simulink model "BFE_TestHarness"  (Simulink 8.6)
settings: Solver=FixedStepDiscrete  StartTime=0.0  StopTime=3  FixedStep=Ts  RelTol=1e-3
PreLoadFcn:
  | addpath('MBD_Tests')
  | 
  | load('Workspace\EnvVar.mat')
  | run('MBD_Tests\MBD_tests_init.m')
  | if exist('tl_preloadfcn','file'), tl_preloadfcn(gcs,402); end
PostLoadFcn:
  | if exist('tl_postloadfcn','file'), tl_postloadfcn(gcs,402); end
InitFcn:
  | if exist('tlds_init','file'), tlds_init(gcs); end
StartFcn:
  | if exist('tlds_start','file'), tlds_start(gcs); end
StopFcn:
  | if exist('tlds_stop','file'), tlds_stop(gcs); end
undefined symbols (not defined in the file): ddv, Ts, u2, u3, u4
libraries: tllib x11, simulink x8, LIB_TF_G_111 x2, LIB_TF_G_12_StepControl x2, LIB_TF_G_112 x1, LIB_TF_G_113 x1
(part 4 of 17)

== system BFE_TestHarness/BFE_AC_BeltFunctionExecution/Subsystem/BFE_AC_BeltFunctionExecution/BFE_AC_BeltFunctionExecution/BFE_runExecuteEmergencyBrakingSequence/Idle State ==
  s16MotorPowerOrder : Inport
  Action Port : ActionPort  ActionType=else
  BFE_MIL_MBD : Constant  RequirementInfo={} %GIDa_d04f2b34_a89a_4659_8327_de322dda7124  Value=ddv('BFE/BFE_MIL_MBD')  mask(TL_Constant){data={'output',{'variable','BFE/BFE_MIL_MBD'},'date',735951.66860642366}}
      settings: CopyFcn=if exist('tl_reset_reviewflag','file')==2,tl_reset_reviewflag(gcbh);end  DeleteFcn=if exist('delete_tlblock','file')==2,delete_tlblock(gcbh);end  NameChangeFcn=if exist('rename_tlblock','file')==2,rename_tlblock(gcbh);end  OpenFcn=if exist('tl_open_blockdlg','file')==2,tl_open_blockdlg(gcbh);else,open_system(gcbh,'parameter');end
      mask Help: eval(['if exist(''tl_online_help'',''file'') == 2, tl_online_help(''Topic'',''TL_Constant''),else, web([''jar:file:///'',matlabroot,''/help/toolbox/simulink/help.jar!/slref/' lower(get_param(gcbh,'Blocktype')) '.html''], ''-helpbrowser''),end'])
      mask Display: plot([-0.05, 1.05, NaN, -0.05, 1.05],[.01, .01, NaN, .99, .99])
  BusCreator : BusCreator  Inputs=2
  Constant : Constant  Value=256  OutDataTypeStr=int16  mask(TL_Constant){data={'date',735951.66860605322}}
      settings: CopyFcn=if exist('tl_reset_reviewflag','file')==2,tl_reset_reviewflag(gcbh);end  DeleteFcn=if exist('delete_tlblock','file')==2,delete_tlblock(gcbh);end  NameChangeFcn=if exist('rename_tlblock','file')==2,rename_tlblock(gcbh);end  OpenFcn=if exist('tl_open_blockdlg','file')==2,tl_open_blockdlg(gcbh);else,open_system(gcbh,'parameter');end
      mask Help: eval(['if exist(''tl_online_help'',''file'') == 2, tl_online_help(''Topic'',''TL_Constant''),else, web([''jar:file:///'',matlabroot,''/help/toolbox/simulink/help.jar!/slref/' lower(get_param(gcbh,'Blocktype')) '.html''], ''-helpbrowser''),end'])
      mask Display: plot([-0.05, 1.05, NaN, -0.05, 1.05],[.01, .01, NaN, .99, .99])
  Data Type Conversion : DataTypeConversion
  If Action Subsystem : Subsystem  RequirementInfo={} %GIDa_d4ad1bcd_a704_4ece_a76e_501b1194cc02  TreatAsAtomicUnit=on
  KUC_ZERO1 : Constant  RequirementInfo={} %GIDa_d1c1a169_18d8_4d2e_970c_33d0bcd7c074  Value=ddv('Common/KU16_ZERO')  mask(TL_Constant){data={'output',{'variable','Common/KU16_ZERO'},'date',735951.66860510421}}
      settings: CopyFcn=if exist('tl_reset_reviewflag','file')==2,tl_reset_reviewflag(gcbh);end  DeleteFcn=if exist('delete_tlblock','file')==2,delete_tlblock(gcbh);end  NameChangeFcn=if exist('rename_tlblock','file')==2,rename_tlblock(gcbh);end  OpenFcn=if exist('tl_open_blockdlg','file')==2,tl_open_blockdlg(gcbh);else,open_system(gcbh,'parameter');end
      mask Help: eval(['if exist(''tl_online_help'',''file'') == 2, tl_online_help(''Topic'',''TL_Constant''),else, web([''jar:file:///'',matlabroot,''/help/toolbox/simulink/help.jar!/slref/' lower(get_param(gcbh,'Blocktype')) '.html''], ''-helpbrowser''),end'])
      mask Display: plot([-0.05, 1.05, NaN, -0.05, 1.05],[.01, .01, NaN, .99, .99])
  Preprocessor IF : If  RequirementInfo={} %GIDa_7af2dae5_defd_43bb_b43b_d22b8c3639ae  IfExpression=u1  ShowElse=off  mask(TL_PreProcessorIf){data={'mode',2,'date',735951.6686047801}}
      settings: DeleteFcn=if exist('delete_tlblock','file')==2,delete_tlblock(gcbh);end  NameChangeFcn=if exist('rename_tlblock','file')==2,rename_tlblock(gcbh);end  OpenFcn=if exist('tl_open_blockdlg','file')==2,tl_open_blockdlg(gcbh);else,open_system(gcbh,'parameter');end
      mask Help: eval(['if exist(''tl_online_help'',''file'') == 2, tl_online_help(''Topic'',''TL_PreProcessorIf''),else, web([''jar:file:///'',matlabroot,''/help/toolbox/simulink/help.jar!/slref/' lower(get_param(gcbh,'Blocktype')) '.html''], ''-helpbrowser''),end'])
      mask Display:
      | plot([-0.05, 1.05, NaN, -0.05, 1.05],[.01, .01, NaN, .99, .99])
      | 
      | port_label('input', 1, 'u1')
      | port_label('output',1,'#ifdef u1');
  Saturation : Saturate  UpperLimit=ddv('Common/KS16_ZERO')  LowerLimit=ddv('BFE/KS16_PWM_MIN_BTN')  mask(TL_Saturate){data={'output',{'name','s16SaturatedPowerOrder'},'lowerlimit',{'variable','BFE/KS16_PWM_MIN_BTN'},'upperlimit',{'variable','Common/KS16_ZERO'},'date',735951.66860453703}}
      settings: CopyFcn=if exist('tl_reset_reviewflag','file')==2,tl_reset_reviewflag(gcbh);end  DeleteFcn=if exist('delete_tlblock','file')==2,delete_tlblock(gcbh);end  NameChangeFcn=if exist('rename_tlblock','file')==2,rename_tlblock(gcbh);end  OpenFcn=if exist('tl_open_blockdlg','file')==2,tl_open_blockdlg(gcbh);else,open_system(gcbh,'parameter');end
      mask Help: eval(['if exist(''tl_online_help'',''file'') == 2, tl_online_help(''Topic'',''TL_Saturate''),else, web([''jar:file:///'',matlabroot,''/help/toolbox/simulink/help.jar!/slref/' lower(get_param(gcbh,'Blocktype')) '.html''], ''-helpbrowser''),end'])
      mask Display: plot([-0.05, 1.05, NaN, -0.05, 1.05],[.01, .01, NaN, .99, .99])
  Src : Subsystem
  Sum : Sum  mask(TL_Sum){data={'output',{'name','s16UnstaturatedPowerOrder'},'date',735951.66860350699}}
      settings: CopyFcn=if exist('tl_reset_reviewflag','file')==2,tl_reset_reviewflag(gcbh);end  DeleteFcn=if exist('delete_tlblock','file')==2,delete_tlblock(gcbh);end  NameChangeFcn=if exist('rename_tlblock','file')==2,rename_tlblock(gcbh);end  OpenFcn=if exist('tl_open_blockdlg','file')==2,tl_open_blockdlg(gcbh);else,open_system(gcbh,'parameter');end
      mask Help: eval(['if exist(''tl_online_help'',''file'') == 2, tl_online_help(''Topic'',''TL_Sum''),else, web([''jar:file:///'',matlabroot,''/help/toolbox/simulink/help.jar!/slref/' lower(get_param(gcbh,'Blocktype')) '.html''], ''-helpbrowser''),end'])
      mask Display: plot([-0.05, 1.05, NaN, -0.05, 1.05],[.01, .01, NaN, .99, .99])
  SSCP_pclMotorPowerOrder_SetPowerOrder : Outport  mask(TL_BusOutport){data={'#autoscaling',2,'#message',2,'#output',2,'#logdata',2,'signals',{{'',{'s16MotorPowerOrder';'u16BoostDutyCycle'}}},'autosar',{'useautosarcommunication',1,'kind',4,'clientserverport','pclMotor_P','operation','SetPowerOrder'},'date',736301.71276452544}}
      settings: CopyFcn=if exist('tl_reset_reviewflag','file')==2,tl_reset_reviewflag(gcbh);end  DeleteFcn=if exist('delete_tlblock','file')==2,delete_tlblock(gcbh);end  NameChangeFcn=if exist('rename_tlblock','file')==2,rename_tlblock(gcbh);end  OpenFcn=if exist('tl_open_blockdlg','file')==2,tl_open_blockdlg(gcbh);else,open_system(gcbh,'parameter');end
      mask Help: eval(['if exist(''tl_online_help'',''file'') == 2, tl_online_help(''Topic'',''TL_Outport''),else, web([''jar:file:///'',matlabroot,''/help/toolbox/simulink/help.jar!/slref/' lower(get_param(gcbh,'Blocktype')) '.html''], ''-helpbrowser''),end'])
      mask Display: plot([0.2 0.35 NaN 0.65 0.8],[0 1 NaN 0 1]);
  s16MotorPowerOrder1 : Outport  Port=2  PortDimensions=1  mask(TL_Outport){data={'autosar',{'useautosarcommunication',1,'kind',3,'communicationmode',1,'interrunnablevariable','s16MotorPowerOrder'},'date',736809.44014694449}}
      settings: CopyFcn=if exist('tl_reset_reviewflag','file')==2,tl_reset_reviewflag(gcbh);end  DeleteFcn=if exist('delete_tlblock','file')==2,delete_tlblock(gcbh);end  NameChangeFcn=if exist('rename_tlblock','file')==2,rename_tlblock(gcbh);end  OpenFcn=if exist('tl_open_blockdlg','file')==2,tl_open_blockdlg(gcbh);else,open_system(gcbh,'parameter');end
      mask Help: eval(['if exist(''tl_online_help'',''file'') == 2, tl_online_help(''Topic'',''TL_Outport''),else, web([''jar:file:///'',matlabroot,''/help/toolbox/simulink/help.jar!/slref/' lower(get_param(gcbh,'Blocktype')) '.html''], ''-helpbrowser''),end'])
      mask Display: plot([0.2 0.35 NaN 0.65 0.8],[0 1 NaN 0 1]);
  u8MotorStageStatus1 : Outport  Port=3  InitialOutput=170
  wires:
  Saturation/1 -> s16MotorPowerOrder1/1, If Action Subsystem/1(MotorPowerOrder), BusCreator/1  "s16MotorPowerOrder"
  KUC_ZERO1/1 -> Data Type Conversion/1  "u16BoostDutyCycle"
  BusCreator/1 -> SSCP_pclMotorPowerOrder_SetPowerOrder/1
  s16MotorPowerOrder/1 -> Sum/1
  Constant/1 -> Sum/2
  Sum/1 -> Saturation/1  "s16MotorPowerOrder"
  Preprocessor IF/1 -> If Action Subsystem/Action
  BFE_MIL_MBD/1 -> Preprocessor IF/1
  Data Type Conversion/1 -> If Action Subsystem/2(BoostPowerOrder), BusCreator/2  "u16BoostDutyCycle"
  Src/1(u8MotorStageStatus) -> u8MotorStageStatus1/1

== system BFE_TestHarness/BFE_AC_BeltFunctionExecution/Subsystem/BFE_AC_BeltFunctionExecution/BFE_AC_BeltFunctionExecution/BFE_runExecuteHighPowerStep/HP feature activated ==
  u16BatteryVoltage : Inport  RequirementInfo={} %GIDa_9f4c284f_e5e1_4494_893c_769a60f6da9b
  u8OrderType : Inport  RequirementInfo={} %GIDa_9ede59d1_628e_47a7_abf0_69ad9a78e7f2  Port=2  OutDataTypeStr=uint8
  s16MotorPowerOrder : Inport  RequirementInfo={} %GIDa_fb0480b8_3596_439f_934a_674bb7f448bd  Port=3
  u32MotorCurrentInmA : Inport  RequirementInfo={} %GIDa_ec4d682a_15d7_421f_80f7_bf84008d9a13  Port=4
  s32FirstOrderValue : Inport  RequirementInfo={} %GIDa_e3027700_74e1_41e6_bdef_dd55c37c19a6  Port=5
  u16StepDuration : Inport  RequirementInfo={} %GIDa_7d66a015_cc67_4524_827e_2d2edff78b49  Port=6
  Action Port : ActionPort  ActionType=then
  Bitwise Operator1 : tllib/Bitwise Operator  RequirementInfo={} %GIDa_d3968feb_3140_49e4_8142_eece2ac41e8b  logicop=AND  UseBitMask=off  NumInputPorts=2  BitMask=bin2dec('11011001')  BitMaskRealWorld=Stored Integer  data={'date',735951.66858835646}
  CurrentRegulation : Subsystem  RequirementInfo={} %GIDa_df169873_29da_4f6f_97c3_f90618a72490  TreatAsAtomicUnit=on
  If : If  RequirementInfo={} %GIDa_a8c59d67_a071_4758_8a53_3fffb38267ab  IfExpression=u1 ~= 0  ShowElse=off
  IsNewCycle : Subsystem  RequirementInfo={} %GIDa_4aa99058_12a3_4b0f_b4dc_b37d50321c32
  KU8_ORDER_HIGH_POWER : Constant  RequirementInfo={} %GIDa_74326903_2aff_476b_98b2_2fe81d9140ab  Value=ddv('RTE_Define/KU8_ORDER_HIGH_POWER')  OutDataTypeStr=uint8  mask(TL_Constant){data={'output',{'variable','RTE_Define/KU8_ORDER_HIGH_POWER'},'date',735951.66841310181}}
      settings: CopyFcn=if exist('tl_reset_reviewflag','file')==2,tl_reset_reviewflag(gcbh);end  DeleteFcn=if exist('delete_tlblock','file')==2,delete_tlblock(gcbh);end  NameChangeFcn=if exist('rename_tlblock','file')==2,rename_tlblock(gcbh);end  OpenFcn=if exist('tl_open_blockdlg','file')==2,tl_open_blockdlg(gcbh);else,open_system(gcbh,'parameter');end
      mask Help: eval(['if exist(''tl_online_help'',''file'') == 2, tl_online_help(''Topic'',''TL_Constant''),else, web([''jar:file:///'',matlabroot,''/help/toolbox/simulink/help.jar!/slref/' lower(get_param(gcbh,'Blocktype')) '.html''], ''-helpbrowser''),end'])
      mask Display: plot([-0.05, 1.05, NaN, -0.05, 1.05],[.01, .01, NaN, .99, .99])
  Relational Operator1 : RelationalOperator  RequirementInfo={} %GIDa_923b10b0_6a02_4409_88e8_7504f8ade75f  Operator=~=  OutDataTypeStr=boolean  mask(TL_RelationalOperator){data={'output',{'name','bIsNewStep'},'date',735951.66841274302}}
      settings: DeleteFcn=if exist('delete_tlblock','file')==2,delete_tlblock(gcbh);end  NameChangeFcn=if exist('rename_tlblock','file')==2,rename_tlblock(gcbh);end  OpenFcn=if exist('tl_open_blockdlg','file')==2,tl_open_blockdlg(gcbh);else,open_system(gcbh,'parameter');end
      mask Help: eval(['if exist(''tl_online_help'',''file'') == 2, tl_online_help(''Topic'',''TL_RelationalOperator''),else, web([''jar:file:///'',matlabroot,''/help/toolbox/simulink/help.jar!/slref/' lower(get_param(gcbh,'Blocktype')) '.html''], ''-helpbrowser''),end'])
      mask Display: plot([-0.05, 1.05, NaN, -0.05, 1.05],[.01, .01, NaN, .99, .99])
  Rescaler : DataTypeConversion  RequirementInfo={} %GIDa_72de47c7_099f_4155_ab0e_4d3f4aead57e  OutDataTypeStr=uint8  SaturateOnIntegerOverflow=on  RndMeth=Zero  mask(TL_Rescaler){data={'output',{'type','UInt8'},'date',735951.66841248842}}
      settings: DeleteFcn=if exist('delete_tlblock','file')==2,delete_tlblock(gcbh);end  NameChangeFcn=if exist('rename_tlblock','file')==2,rename_tlblock(gcbh);end  OpenFcn=if exist('tl_open_blockdlg','file')==2,tl_open_blockdlg(gcbh);else,open_system(gcbh,'parameter');end
      mask Help: eval(['if exist(''tl_online_help'',''file'') == 2, tl_online_help(''Topic'',''TL_Rescaler''),else, web([''jar:file:///'',matlabroot,''/help/toolbox/simulink/help.jar!/slref/' lower(get_param(gcbh,'Blocktype')) '.html''], ''-helpbrowser''),end'])
      mask Display: plot([-0.05, 1.05, NaN, -0.05, 1.05],[.01, .01, NaN, .99, .99])
  Terminator : Terminator
      settings: RequirementInfo={} %GIDa_1a576c7a_f67d_44a4_8373_5dddf82b8885
  Terminator1 : Terminator
      settings: RequirementInfo={} %GIDa_adf98c52_d575_4689_a55b_9bedd9a0bfd9
  Unit Delay2 : UnitDelay  RequirementInfo={} %GIDa_03689cc4_3b49_4537_8280_a158703a02cf  SampleTime=-1  mask(TL_UnitDelay){data={'output',{'type','Int32'},'state',{'name','s32OldFirstOrderValue','type','Int32'},'date',735951.66841215279}}
      settings: CopyFcn=if exist('tl_reset_reviewflag','file')==2,tl_reset_reviewflag(gcbh);end  DeleteFcn=if exist('delete_tlblock','file')==2,delete_tlblock(gcbh);end  NameChangeFcn=if exist('rename_tlblock','file')==2,rename_tlblock(gcbh);end  OpenFcn=if exist('tl_open_blockdlg','file')==2,tl_open_blockdlg(gcbh);else,open_system(gcbh,'parameter');end
      mask Help: eval(['if exist(''tl_online_help'',''file'') == 2, tl_online_help(''Topic'',''TL_UnitDelay''),else, web([''jar:file:///'',matlabroot,''/help/toolbox/simulink/help.jar!/slref/' lower(get_param(gcbh,'Blocktype')) '.html''], ''-helpbrowser''),end'])
      mask Display: plot([-0.05, 1.05, NaN, -0.05, 1.05],[.01, .01, NaN, .99, .99])
  wires:
  If/1 -> CurrentRegulation/Action
  s32FirstOrderValue/1 -> CurrentRegulation/5(s32FirstOrderValue), Relational Operator1/1, Unit Delay2/1
  s16MotorPowerOrder/1 -> CurrentRegulation/3(MotorSign)
  u32MotorCurrentInmA/1 -> CurrentRegulation/4(ReadMotorCurrentInmA)
  Bitwise Operator1/1 -> If/1
  u8OrderType/1 -> IsNewCycle/1(u8OrderType), Rescaler/1
  u16BatteryVoltage/1 -> CurrentRegulation/2(u16BatteryVoltage)
  u16StepDuration/1 -> CurrentRegulation/6(u16StepDuration)
  Unit Delay2/1 -> Relational Operator1/2
  Relational Operator1/1 -> CurrentRegulation/7(IsNewStep)
  IsNewCycle/1(IsNewCycle) -> CurrentRegulation/1(IsNewCycle)
  KU8_ORDER_HIGH_POWER/1 -> Bitwise Operator1/1
  Rescaler/1 -> Bitwise Operator1/2
  CurrentRegulation/1(SSCP_pclMotorPowerOrder_SetPowerOrder) -> Terminator/1
  CurrentRegulation/2(s16MotorPowerOrder1) -> Terminator1/1

== system BFE_TestHarness/BFE_AC_BeltFunctionExecution/Subsystem/BFE_AC_BeltFunctionExecution/BFE_AC_BeltFunctionExecution/BFE_runExecuteStandardSteps/ExecuteStandardSteps ==
  OA_pclVehicleAnalogSignals_GetBatteryVoltage : Inport  RequirementInfo={} %GIDa_38d80fb2_8518_431e_9df3_31d74e981ccc  OutDataTypeStr=uint16
  OA_pclMotorCurrent_ReadMotorCurrentInmA : Inport  RequirementInfo={} %GIDa_d42d6ad4_2d69_4f86_a4d4_8d1cf902a910  Port=2
  u8OrderType : Inport  RequirementInfo={} %GIDa_17864709_fab6_441f_9427_1627f567cba4  Port=3
  s32FirstOrderValue : Inport  RequirementInfo={} %GIDa_56d0bdfd_bbb3_41b1_980b_3ae94e95e045  Port=4
  s32OrderIncrementValue : Inport  RequirementInfo={} %GIDa_c9367d53_d735_49a0_b5e8_7dead65c6176  Port=5
  s16OldPwm : Inport  RequirementInfo={} %GIDa_1e269e6c_84ef_43a4_b67f_2684ba3d7e58  Port=6  OutDataTypeStr=int16
  bIsPrevStepHP : Inport  RequirementInfo={} %GIDa_bc912459_a8ca_4020_ada6_c2822196c8bb  Port=7  OutDataTypeStr=uint8
  u8MotorStageStatus : Inport  Port=8
  Action Port : ActionPort  RequirementInfo={} %GIDa_709d0def_6123_428f_8adf_681e6886f8b2  ActionType=then
  Abs : Abs  mask(TL_Abs){data={'output',{'name','u32AbsMotorCurrent','type','UInt32'},'date',735951.66840594902}}
      settings: CopyFcn=if exist('tl_reset_reviewflag','file')==2,tl_reset_reviewflag(gcbh);end  DeleteFcn=if exist('delete_tlblock','file')==2,delete_tlblock(gcbh);end  NameChangeFcn=if exist('rename_tlblock','file')==2,rename_tlblock(gcbh);end  OpenFcn=if exist('tl_open_blockdlg','file')==2,tl_open_blockdlg(gcbh);else,open_system(gcbh,'parameter');end
      mask Help: eval(['if exist(''tl_online_help'',''file'') == 2, tl_online_help(''Topic'',''TL_Abs''),else, web([''jar:file:///'',matlabroot,''/help/toolbox/simulink/help.jar!/slref/' lower(get_param(gcbh,'Blocktype')) '.html''], ''-helpbrowser''),end'])
      mask Display: plot([-0.05, 1.05, NaN, -0.05, 1.05],[.01, .01, NaN, .99, .99])
  Mange Power Stage consign update : Subsystem  TreatAsAtomicUnit=on
  Saturation : Saturate  RequirementInfo={} %GIDa_bc6cb916_2c6b_4c0f_aef7_8e292914ffe4  UpperLimit=ddv('BFE/KS16_PWM_MAX_BTN')  LowerLimit=ddv('BFE/KS16_PWM_MIN_BTN')  OutDataTypeStr=int16  mask(TL_Saturate){data={'lowerlimit',{'variable','BFE/KS16_PWM_MIN_BTN'},'upperlimit',{'variable','BFE/KS16_PWM_MAX_BTN'},'date',735951.66839928238}}
      settings: CopyFcn=if exist('tl_reset_reviewflag','file')==2,tl_reset_reviewflag(gcbh);end  DeleteFcn=if exist('delete_tlblock','file')==2,delete_tlblock(gcbh);end  NameChangeFcn=if exist('rename_tlblock','file')==2,rename_tlblock(gcbh);end  OpenFcn=if exist('tl_open_blockdlg','file')==2,tl_open_blockdlg(gcbh);else,open_system(gcbh,'parameter');end
      mask Help: eval(['if exist(''tl_online_help'',''file'') == 2, tl_online_help(''Topic'',''TL_Saturate''),else, web([''jar:file:///'',matlabroot,''/help/toolbox/simulink/help.jar!/slref/' lower(get_param(gcbh,'Blocktype')) '.html''], ''-helpbrowser''),end'])
      mask Display: plot([-0.05, 1.05, NaN, -0.05, 1.05],[.01, .01, NaN, .99, .99])
  SubsystemConvertOrderToMotorPower : Subsystem  RequirementInfo={} %GIDa_bcaf6223_33b1_4352_bc9f_73984f09d03f
  SubsystemUpdateConsigns : Subsystem  RequirementInfo={} %GIDa_8132c1ce_d6cc_4edb_bd84_e1aba50faacc
  Terminator : Terminator
      settings: RequirementInfo={} %GIDa_3ae8cfeb_ade5_402f_93e0_64b114af98cc
  Terminator1 : Terminator
      settings: RequirementInfo={} %GIDa_57c8c38c_f0c0_45fc_878f_e394488758fb
  wires:
  s32OrderIncrementValue/1 -> SubsystemUpdateConsigns/1(lMilliOrderIncrement)
  s32FirstOrderValue/1 -> SubsystemUpdateConsigns/2(lMilliOrder)
  u8OrderType/1 -> SubsystemConvertOrderToMotorPower/1(u8OrderType)
  SubsystemUpdateConsigns/1(bAreConsignsChanged) -> SubsystemConvertOrderToMotorPower/2(bIsNewStepBegin)
  SubsystemUpdateConsigns/2(lOrderToApply) -> SubsystemConvertOrderToMotorPower/3(s32OrderToApply)
  OA_pclVehicleAnalogSignals_GetBatteryVoltage/1 -> SubsystemConvertOrderToMotorPower/4(u16BatteryVoltage)
  OA_pclMotorCurrent_ReadMotorCurrentInmA/1 -> Abs/1
  SubsystemConvertOrderToMotorPower/1(s16UnsaturatedMotorPower) -> Saturation/1
  Saturation/1 -> Mange Power Stage consign update/2(In1)  "s16MotorPowerOrder"
  s16OldPwm/1 -> SubsystemConvertOrderToMotorPower/6(s8OldPwm)
  bIsPrevStepHP/1 -> SubsystemConvertOrderToMotorPower/7(bIsPrevStepHP)
  u8MotorStageStatus/1 -> Mange Power Stage consign update/1(u8MotorStageStatus)
  Mange Power Stage consign update/1(SSCP_pclMotorPowerOrder_SetPowerOrder) -> Terminator/1
  Mange Power Stage consign update/2(s16MotorPowerOrder1) -> Terminator1/1
  Abs/1 -> SubsystemConvertOrderToMotorPower/5(u32MeasuredCurrent)

== system BFE_TestHarness/BFE_AC_BeltFunctionExecution/Subsystem/BFE_AC_BeltFunctionExecution/BFE_AC_BeltFunctionExecution/BFE_runResetMotorStageStatus/Src ==
  Const : Constant  Value=ddv('RTE_Define/KU8_MOTOR_STAGE_ACTIVATION')  mask(TL_Constant){data={'output',{'variable','RTE_Define/KU8_MOTOR_STAGE_ACTIVATION'},'date',735951.66850025463}}
      settings: CopyFcn=if exist('tl_reset_reviewflag','file')==2,tl_reset_reviewflag(gcbh);end  DeleteFcn=if exist('delete_tlblock','file')==2,delete_tlblock(gcbh);end  NameChangeFcn=if exist('rename_tlblock','file')==2,rename_tlblock(gcbh);end  OpenFcn=if exist('tl_open_blockdlg','file')==2,tl_open_blockdlg(gcbh);else,open_system(gcbh,'parameter');end
      mask Help: eval(['if exist(''tl_online_help'',''file'') == 2, tl_online_help(''Topic'',''TL_Constant''),else, web([''jar:file:///'',matlabroot,''/help/toolbox/simulink/help.jar!/slref/' lower(get_param(gcbh,'Blocktype')) '.html''], ''-helpbrowser''),end'])
      mask Display: plot([-0.05, 1.05, NaN, -0.05, 1.05],[.01, .01, NaN, .99, .99])
  u8MotorStageStatus : Outport
  wires:
  Const/1 -> u8MotorStageStatus/1  "u8MotorStageStatus"

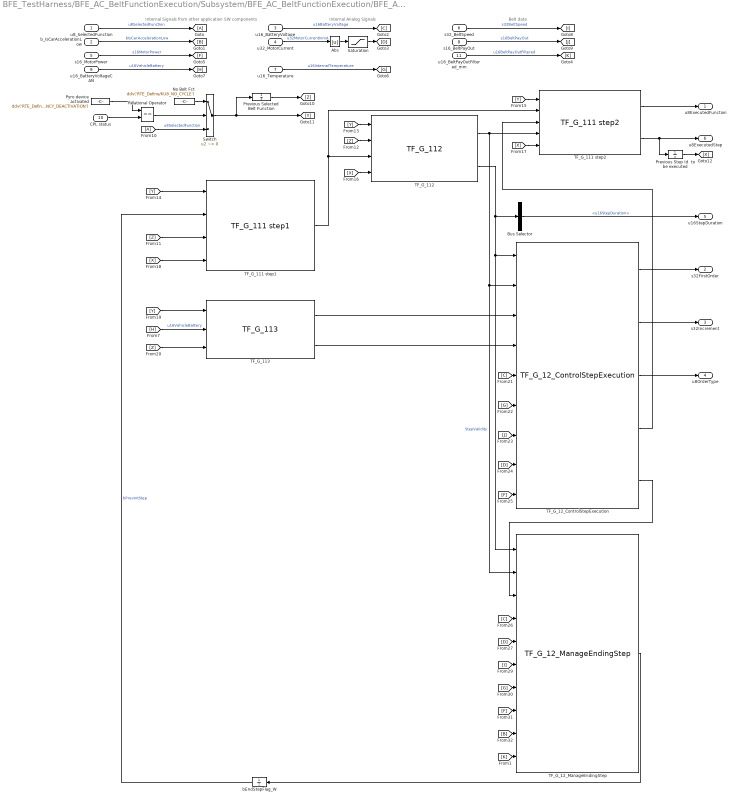
== system BFE_TestHarness/BFE_AC_BeltFunctionExecution/Subsystem/BFE_AC_BeltFunctionExecution/BFE_AC_BeltFunctionExecution/BFE_runScheduleStep/BFE_Core ==
  note: Internal Analog Signals
  note: Internal Signals from other application SW components
  note: Belt data
  u8_SelectedFunction : Inport  RequirementInfo={} %GIDa_0942ee6a_5c2c_4c70_b0cb_396269c7c0d7  OutDataTypeStr=uint8
  b_IsCarAccelerationLow : Inport  RequirementInfo={} %GIDa_d98bb0b4_4728_4521_8742_e5779416ddf8  Port=2
  u16_BatteryVoltage : Inport  RequirementInfo={} %GIDa_394494ec_7aac_4638_9330_05024365204b  Port=3
  u32_MotorCurrent : Inport  RequirementInfo={} %GIDa_6085fdc7_666f_447a_8bec_7e89f698cd05  Port=4
  s16_MotorPower : Inport  RequirementInfo={} %GIDa_4a5abf86_670e_4c15_b3fe_a5ee2ba10c03  Port=5  OutDataTypeStr=int16
  s32_BeltSpeed : Inport  RequirementInfo={} %GIDa_a8012ebd_3dd5_4348_80d5_6693b3966d38  Port=6
  u16_Temperature : Inport  RequirementInfo={} %GIDa_74dc6bf2_9f78_4341_87c4_124b718df474  Port=7  OutDataTypeStr=uint16
  s16_BeltPayOut : Inport  RequirementInfo={} %GIDa_5a9f3083_1bb9_4a9b_84ba_7c6521c988e0  Port=8  OutDataTypeStr=int16
  u16_BatteryVoltageCAN : Inport  RequirementInfo={} %GIDa_ea72efb0_a669_4c6f_a141_7d1891d9e8e1  Port=9
  CPL status : Inport  Port=10
  u16_BeltPayOutFiltered_mm : Inport  RequirementInfo={} %GIDa_81b28c81_e017_48a4_977b_234887a600f0  Port=11  OutDataTypeStr=uint16
  Abs : Abs  mask(TL_Abs){data={'output',{'type','UInt32'},'date',735951.66849038191}}
      settings: CopyFcn=if exist('tl_reset_reviewflag','file')==2,tl_reset_reviewflag(gcbh);end  DeleteFcn=if exist('delete_tlblock','file')==2,delete_tlblock(gcbh);end  NameChangeFcn=if exist('rename_tlblock','file')==2,rename_tlblock(gcbh);end  OpenFcn=if exist('tl_open_blockdlg','file')==2,tl_open_blockdlg(gcbh);else,open_system(gcbh,'parameter');end
      mask Help: eval(['if exist(''tl_online_help'',''file'') == 2, tl_online_help(''Topic'',''TL_Abs''),else, web([''jar:file:///'',matlabroot,''/help/toolbox/simulink/help.jar!/slref/' lower(get_param(gcbh,'Blocktype')) '.html''], ''-helpbrowser''),end'])
      mask Display: plot([-0.05, 1.05, NaN, -0.05, 1.05],[.01, .01, NaN, .99, .99])
  Bus Selector : BusSelector  OutputSignals=u16StepDuration
  No Belt Fct : Constant  Value=ddv('RTE_Define/KU8_NO_CYCLE')  mask(TL_Constant){data={'output',{'variable','RTE_Define/KU8_NO_CYCLE'},'date',735951.66849003476}}
      settings: CopyFcn=if exist('tl_reset_reviewflag','file')==2,tl_reset_reviewflag(gcbh);end  DeleteFcn=if exist('delete_tlblock','file')==2,delete_tlblock(gcbh);end  NameChangeFcn=if exist('rename_tlblock','file')==2,rename_tlblock(gcbh);end  OpenFcn=if exist('tl_open_blockdlg','file')==2,tl_open_blockdlg(gcbh);else,open_system(gcbh,'parameter');end
      mask Help: eval(['if exist(''tl_online_help'',''file'') == 2, tl_online_help(''Topic'',''TL_Constant''),else, web([''jar:file:///'',matlabroot,''/help/toolbox/simulink/help.jar!/slref/' lower(get_param(gcbh,'Blocktype')) '.html''], ''-helpbrowser''),end'])
      mask Display: plot([-0.05, 1.05, NaN, -0.05, 1.05],[.01, .01, NaN, .99, .99])
  Previous Selected Belt Function : UnitDelay  InitialCondition=255  SampleTime=-1  mask(TL_UnitDelay){data={'output',{'type','UInt8'},'state',{'name','u8PreviousSelectedCycle','type','UInt8'},'date',735951.66848964116}}
      settings: CopyFcn=if exist('tl_reset_reviewflag','file')==2,tl_reset_reviewflag(gcbh);end  DeleteFcn=if exist('delete_tlblock','file')==2,delete_tlblock(gcbh);end  NameChangeFcn=if exist('rename_tlblock','file')==2,rename_tlblock(gcbh);end  OpenFcn=if exist('tl_open_blockdlg','file')==2,tl_open_blockdlg(gcbh);else,open_system(gcbh,'parameter');end
      mask Help: eval(['if exist(''tl_online_help'',''file'') == 2, tl_online_help(''Topic'',''TL_UnitDelay''),else, web([''jar:file:///'',matlabroot,''/help/toolbox/simulink/help.jar!/slref/' lower(get_param(gcbh,'Blocktype')) '.html''], ''-helpbrowser''),end'])
      mask Display: plot([-0.05, 1.05, NaN, -0.05, 1.05],[.01, .01, NaN, .99, .99])
  Previous Step Id  to be executed : UnitDelay  RequirementInfo={} %GIDa_474cf706_01ee_436e_9808_ee5977b68313  InitialCondition=ddv('BFE/KUC_UNDEFINED_STEP')  SampleTime=-1  mask(TL_UnitDelay){data={'output',{'type','UInt8'},'state',{'name','u8PreviousStepToExecute','type','UInt8'},'date',735951.66848909727}}
      settings: CopyFcn=if exist('tl_reset_reviewflag','file')==2,tl_reset_reviewflag(gcbh);end  DeleteFcn=if exist('delete_tlblock','file')==2,delete_tlblock(gcbh);end  NameChangeFcn=if exist('rename_tlblock','file')==2,rename_tlblock(gcbh);end  OpenFcn=if exist('tl_open_blockdlg','file')==2,tl_open_blockdlg(gcbh);else,open_system(gcbh,'parameter');end
      mask Help: eval(['if exist(''tl_online_help'',''file'') == 2, tl_online_help(''Topic'',''TL_UnitDelay''),else, web([''jar:file:///'',matlabroot,''/help/toolbox/simulink/help.jar!/slref/' lower(get_param(gcbh,'Blocktype')) '.html''], ''-helpbrowser''),end'])
      mask Display: plot([-0.05, 1.05, NaN, -0.05, 1.05],[.01, .01, NaN, .99, .99])
  Pyro device activated : Constant  Value=ddv('RTE_Define/KU8_MOTOR_STAGE_EMERGENCY_DEACTIVATION')  mask(TL_Constant){data={'output',{'variable','RTE_Define/KU8_MOTOR_STAGE_EMERGENCY_DEACTIVATION'},'date',735951.66848859959}}
      settings: CopyFcn=if exist('tl_reset_reviewflag','file')==2,tl_reset_reviewflag(gcbh);end  DeleteFcn=if exist('delete_tlblock','file')==2,delete_tlblock(gcbh);end  NameChangeFcn=if exist('rename_tlblock','file')==2,rename_tlblock(gcbh);end  OpenFcn=if exist('tl_open_blockdlg','file')==2,tl_open_blockdlg(gcbh);else,open_system(gcbh,'parameter');end
      mask Help: eval(['if exist(''tl_online_help'',''file'') == 2, tl_online_help(''Topic'',''TL_Constant''),else, web([''jar:file:///'',matlabroot,''/help/toolbox/simulink/help.jar!/slref/' lower(get_param(gcbh,'Blocktype')) '.html''], ''-helpbrowser''),end'])
      mask Display: plot([-0.05, 1.05, NaN, -0.05, 1.05],[.01, .01, NaN, .99, .99])
  Relational Operator : RelationalOperator  Operator===  OutDataTypeStr=boolean  mask(TL_RelationalOperator){data={'date',735951.66848825233}}
      settings: DeleteFcn=if exist('delete_tlblock','file')==2,delete_tlblock(gcbh);end  NameChangeFcn=if exist('rename_tlblock','file')==2,rename_tlblock(gcbh);end  OpenFcn=if exist('tl_open_blockdlg','file')==2,tl_open_blockdlg(gcbh);else,open_system(gcbh,'parameter');end
      mask Help: eval(['if exist(''tl_online_help'',''file'') == 2, tl_online_help(''Topic'',''TL_RelationalOperator''),else, web([''jar:file:///'',matlabroot,''/help/toolbox/simulink/help.jar!/slref/' lower(get_param(gcbh,'Blocktype')) '.html''], ''-helpbrowser''),end'])
      mask Display: plot([-0.05, 1.05, NaN, -0.05, 1.05],[.01, .01, NaN, .99, .99])
  Saturation : Saturate  UpperLimit=100000  LowerLimit=0  mask(TL_Saturate){data={'output',{'name','u32SaturatedMotorCurrent','type','UInt32'},'date',735951.66848793987}}
      settings: CopyFcn=if exist('tl_reset_reviewflag','file')==2,tl_reset_reviewflag(gcbh);end  DeleteFcn=if exist('delete_tlblock','file')==2,delete_tlblock(gcbh);end  NameChangeFcn=if exist('rename_tlblock','file')==2,rename_tlblock(gcbh);end  OpenFcn=if exist('tl_open_blockdlg','file')==2,tl_open_blockdlg(gcbh);else,open_system(gcbh,'parameter');end
      mask Help: eval(['if exist(''tl_online_help'',''file'') == 2, tl_online_help(''Topic'',''TL_Saturate''),else, web([''jar:file:///'',matlabroot,''/help/toolbox/simulink/help.jar!/slref/' lower(get_param(gcbh,'Blocktype')) '.html''], ''-helpbrowser''),end'])
      mask Display: plot([-0.05, 1.05, NaN, -0.05, 1.05],[.01, .01, NaN, .99, .99])
  Switch : Switch  Criteria=u2 ~= 0  mask(TL_Switch){data={'output',{'name','u8FilteredSelectedCycle','type','UInt8'},'date',735951.66848730319}}
      settings: CopyFcn=if exist('tl_reset_reviewflag','file')==2,tl_reset_reviewflag(gcbh);end  DeleteFcn=if exist('delete_tlblock','file')==2,delete_tlblock(gcbh);end  NameChangeFcn=if exist('rename_tlblock','file')==2,rename_tlblock(gcbh);end  OpenFcn=if exist('tl_open_blockdlg','file')==2,tl_open_blockdlg(gcbh);else,open_system(gcbh,'parameter');end
      mask Help: eval(['if exist(''tl_online_help'',''file'') == 2, tl_online_help(''Topic'',''TL_Switch''),else, web([''jar:file:///'',matlabroot,''/help/toolbox/simulink/help.jar!/slref/' lower(get_param(gcbh,'Blocktype')) '.html''], ''-helpbrowser''),end'])
      mask Display: plot([-0.05, 1.05, NaN, -0.05, 1.05],[.01, .01, NaN, .99, .99])
  TF_G_111 step1 : LIB_TF_G_111/TF_G_111 step1  RequirementInfo={} %GIDa_1baf4a10_21df_4359_ba4d_6c5534378a62
  TF_G_111 step2 : LIB_TF_G_111/TF_G_111 step2  Description=The subsystemDetermineExecutedFunction block is in charge of providing the current executed function output.  RequirementInfo={} %GIDa_81c3cd2c_4953_404a_b1b0_29a375d31300
  TF_G_112 : LIB_TF_G_112/TF_G_112
  TF_G_113 : LIB_TF_G_113/TF_G_113
  TF_G_12_ControlStepExecution : LIB_TF_G_12_StepControl/TF_G_12_ControlStepExecution
  TF_G_12_ManageEndingStep : LIB_TF_G_12_StepControl/TF_G_12_ManageEndingStep
  bEndStepFlag_W : UnitDelay  RequirementInfo={} %GIDa_70daf7a2_6375_4b25_a07f_51c1c96c5194  InitialCondition=1  SampleTime=-1  mask(TL_UnitDelay){data={'logdata',{'loggingmode',1},'output',{'type','Bool'},'state',{'name','bOldEndStep','type','Bool'},'date',735951.66845576384}}
      settings: CopyFcn=if exist('tl_reset_reviewflag','file')==2,tl_reset_reviewflag(gcbh);end  DeleteFcn=if exist('delete_tlblock','file')==2,delete_tlblock(gcbh);end  NameChangeFcn=if exist('rename_tlblock','file')==2,rename_tlblock(gcbh);end  OpenFcn=if exist('tl_open_blockdlg','file')==2,tl_open_blockdlg(gcbh);else,open_system(gcbh,'parameter');end
      mask Help: eval(['if exist(''tl_online_help'',''file'') == 2, tl_online_help(''Topic'',''TL_UnitDelay''),else, web([''jar:file:///'',matlabroot,''/help/toolbox/simulink/help.jar!/slref/' lower(get_param(gcbh,'Blocktype')) '.html''], ''-helpbrowser''),end'])
      mask Display: plot([-0.05, 1.05, NaN, -0.05, 1.05],[.01, .01, NaN, .99, .99])
  u8ExecutedFunction : Outport  RequirementInfo={} %GIDa_e291138d_76f0_4298_b8f7_e1cf85ecc9f8
  s32FirstOrder : Outport  RequirementInfo={} %GIDa_d3f3219f_a008_4ad9_a04b_5255231d0ce6  Port=2
  s32Increment : Outport  RequirementInfo={} %GIDa_2d1e5874_67ac_45a3_8209_b547920f8565  Port=3
  u8OrderType : Outport  RequirementInfo={} %GIDa_d191614f_7790_4e22_b3f9_2cfc50774c28  Port=4
  u16StepDuration : Outport  RequirementInfo={} %GIDa_42820dfe_c66a_484b_bd61_e2b89a82e359  Port=5
  u8ExecutedStep : Outport  RequirementInfo={} %GIDa_d95022a3_b617_4e5b_bbeb_17e7c741b91c  Port=6
  wires:
  bEndStepFlag_W/1 -> TF_G_111 step1/2  "bPrevIntStep"
  u8_SelectedFunction/1 -> [A]  "u8SelectedFunction"
  b_IsCarAccelerationLow/1 -> [B]  "bIsCarAccelerationLow"
  u16_BatteryVoltage/1 -> [C]  "u16BatteryVoltage"
  u32_MotorCurrent/1 -> Abs/1  "u32MotorCurrentInmA"
  s16_MotorPower/1 -> [F]  "s16MotorPower"
  u16_Temperature/1 -> [G]  "u16InternalTemperature"
  u16_BatteryVoltageCAN/1 -> [H]  "u16VehicleBattery"
  s32_BeltSpeed/1 -> [I]  "s32BeltSpeed"
  s16_BeltPayOut/1 -> [J]  "s16BeltPayOut"
  [A] -> Switch/3  "u8SelectedFunction"
  CPL status/1 -> Relational Operator/2
  Pyro device activated/1 -> Relational Operator/1
  Relational Operator/1 -> Switch/2
  No Belt Fct/1 -> Switch/1
  Switch/1 -> Previous Selected Belt Function/1, [Y]
  Previous Selected Belt Function/1 -> [Z]
  [Z] -> TF_G_111 step1/3
  TF_G_111 step1/1 -> TF_G_111 step2/2, TF_G_112/3
  TF_G_111 step2/1 -> u8ExecutedFunction/1
  TF_G_111 step2/2 -> u8ExecutedStep/1, Previous Step Id  to be executed/1
  [Z] -> TF_G_112/2
  TF_G_112/1 -> TF_G_111 step2/4, TF_G_12_ControlStepExecution/2, TF_G_12_ManageEndingStep/2  "StepValidity"
  [Y] -> TF_G_112/1
  [Y] -> TF_G_111 step1/1
  [Y] -> TF_G_111 step2/1
  Previous Step Id  to be executed/1 -> [X]
  [X] -> TF_G_112/4
  [X] -> TF_G_111 step2/5
  [X] -> TF_G_111 step1/4
  [Y] -> TF_G_113/1
  [H] -> TF_G_113/2  "u16VehicleBattery"
  [Z] -> TF_G_113/3
  TF_G_113/1 -> TF_G_12_ControlStepExecution/3
  TF_G_113/2 -> TF_G_12_ControlStepExecution/4
  TF_G_112/2 -> Bus Selector/1, TF_G_12_ControlStepExecution/1, TF_G_12_ManageEndingStep/1
  [C] -> TF_G_12_ControlStepExecution/5
  [G] -> TF_G_12_ControlStepExecution/6
  [J] -> TF_G_12_ControlStepExecution/7
  [D] -> TF_G_12_ControlStepExecution/8
  [F] -> TF_G_12_ControlStepExecution/9
  TF_G_12_ControlStepExecution/1 -> s32FirstOrder/1
  TF_G_12_ControlStepExecution/2 -> s32Increment/1
  TF_G_12_ControlStepExecution/3 -> u8OrderType/1
  TF_G_12_ControlStepExecution/4 -> TF_G_111 step2/3
  Bus Selector/1 -> u16StepDuration/1  "<u16StepDuration>"
  TF_G_12_ManageEndingStep/1 -> bEndStepFlag_W/1
  TF_G_12_ControlStepExecution/5 -> TF_G_12_ManageEndingStep/3
  [C] -> TF_G_12_ManageEndingStep/4
  [D] -> TF_G_12_ManageEndingStep/5
  [I] -> TF_G_12_ManageEndingStep/6
  Saturation/1 -> [D]
  Abs/1 -> Saturation/1
  u16_BeltPayOutFiltered_mm/1 -> [K]  "u16BeltPayOutFiltered"
  [G] -> TF_G_12_ManageEndingStep/7
  [F] -> TF_G_12_ManageEndingStep/8
  [B] -> TF_G_12_ManageEndingStep/9
  [K] -> TF_G_12_ManageEndingStep/10

== system BFE_TestHarness/BFE_AC_BeltFunctionExecution/Subsystem/BFE_AC_BeltFunctionExecution/BFE_AC_BeltFunctionExecution/BFE_runScheduleStep/Critical section for outputs to  protect against ISR access ==
  FirstOrder : Inport
  Increment : Inport  Port=2
  OrderType : Inport  Port=3
  Duration : Inport  Port=4
  Demux : Demux
  Function-Call Generator : simulink/Ports & Subsystems/Function-Call Generator  sample_time=-1  numberOfIterations=1
  Switch Case Action Subsystem : Subsystem  TreatAsAtomicUnit=on
  Switch Case Action Subsystem1 : Subsystem  TreatAsAtomicUnit=on
  Switch Case Action Subsystem2 : Subsystem  TreatAsAtomicUnit=on
  Switch Case Action Subsystem3 : Subsystem  TreatAsAtomicUnit=on
  Out_Increment : Outport
  Out_FirstOrder : Outport  Port=2
  Out_Duration : Outport  Port=3
  Out_OrderType : Outport  Port=4
  wires:
  Function-Call Generator/1 -> Demux/1
  Increment/1 -> Switch Case Action Subsystem/1(In1)
  Demux/1 -> Switch Case Action Subsystem/Trigger
  Switch Case Action Subsystem/1(s32OrderIncrementValue) -> Out_Increment/1
  FirstOrder/1 -> Switch Case Action Subsystem1/1(In1)
  Switch Case Action Subsystem1/1(s32FirstOrderValue) -> Out_FirstOrder/1
  Demux/2 -> Switch Case Action Subsystem1/Trigger
  Switch Case Action Subsystem2/1(u16StepDuration) -> Out_Duration/1
  Duration/1 -> Switch Case Action Subsystem2/1(In1)
  Demux/3 -> Switch Case Action Subsystem2/Trigger
  Switch Case Action Subsystem3/1(u8OrderType) -> Out_OrderType/1
  Demux/4 -> Switch Case Action Subsystem3/Trigger
  OrderType/1 -> Switch Case Action Subsystem3/1(In1)

== system BFE_TestHarness/BFE_AC_BeltFunctionExecution/Subsystem/BFE_AC_BeltFunctionExecution/BFE_AC_BeltFunctionExecution/ManageRunnables/If Action Subsystem ==
  Trigger : TriggerPort  RequirementInfo={} %GIDa_d4b65077_5d85_41a2_b0ef_246f62ef6a98  TriggerType=function-call
  Constant : Constant  RequirementInfo={} %GIDa_301442ff_6894_4ca4_93e1_777e7a057398  mask(TL_Constant){data={'date',735951.66844975692}}
      settings: CopyFcn=if exist('tl_reset_reviewflag','file')==2,tl_reset_reviewflag(gcbh);end  DeleteFcn=if exist('delete_tlblock','file')==2,delete_tlblock(gcbh);end  NameChangeFcn=if exist('rename_tlblock','file')==2,rename_tlblock(gcbh);end  OpenFcn=if exist('tl_open_blockdlg','file')==2,tl_open_blockdlg(gcbh);else,open_system(gcbh,'parameter');end
      mask Help: eval(['if exist(''tl_online_help'',''file'') == 2, tl_online_help(''Topic'',''TL_Constant''),else, web([''jar:file:///'',matlabroot,''/help/toolbox/simulink/help.jar!/slref/' lower(get_param(gcbh,'Blocktype')) '.html''], ''-helpbrowser''),end'])
      mask Display: plot([-0.05, 1.05, NaN, -0.05, 1.05],[.01, .01, NaN, .99, .99])
  Constant2 : Constant  RequirementInfo={} %GIDa_f3c71606_bf9d_418f_be49_adf7fd5916df  Value=25  mask(TL_Constant){data={'date',735951.66844939813}}
      settings: CopyFcn=if exist('tl_reset_reviewflag','file')==2,tl_reset_reviewflag(gcbh);end  DeleteFcn=if exist('delete_tlblock','file')==2,delete_tlblock(gcbh);end  NameChangeFcn=if exist('rename_tlblock','file')==2,rename_tlblock(gcbh);end  OpenFcn=if exist('tl_open_blockdlg','file')==2,tl_open_blockdlg(gcbh);else,open_system(gcbh,'parameter');end
      mask Help: eval(['if exist(''tl_online_help'',''file'') == 2, tl_online_help(''Topic'',''TL_Constant''),else, web([''jar:file:///'',matlabroot,''/help/toolbox/simulink/help.jar!/slref/' lower(get_param(gcbh,'Blocktype')) '.html''], ''-helpbrowser''),end'])
      mask Display: plot([-0.05, 1.05, NaN, -0.05, 1.05],[.01, .01, NaN, .99, .99])
  Constant4 : Constant  RequirementInfo={} %GIDa_50c248d0_d58d_4bbd_bf53_b9ea3a2626c5  Value=0  mask(TL_Constant){data={'date',735951.66844902781}}
      settings: CopyFcn=if exist('tl_reset_reviewflag','file')==2,tl_reset_reviewflag(gcbh);end  DeleteFcn=if exist('delete_tlblock','file')==2,delete_tlblock(gcbh);end  NameChangeFcn=if exist('rename_tlblock','file')==2,rename_tlblock(gcbh);end  OpenFcn=if exist('tl_open_blockdlg','file')==2,tl_open_blockdlg(gcbh);else,open_system(gcbh,'parameter');end
      mask Help: eval(['if exist(''tl_online_help'',''file'') == 2, tl_online_help(''Topic'',''TL_Constant''),else, web([''jar:file:///'',matlabroot,''/help/toolbox/simulink/help.jar!/slref/' lower(get_param(gcbh,'Blocktype')) '.html''], ''-helpbrowser''),end'])
      mask Display: plot([-0.05, 1.05, NaN, -0.05, 1.05],[.01, .01, NaN, .99, .99])
  If : If  RequirementInfo={} %GIDa_347c6ffa_a59f_4773_bfe1_c4c7b67e98bd  IfExpression=u1  ShowElse=off
  If Action Subsystem : Subsystem  RequirementInfo={} %GIDa_652e374b_06c1_4dff_9196_3616081d84b9  TreatAsAtomicUnit=on
  Math1 : Math  RequirementInfo={} %GIDa_cff8314e_ca90_4e12_82e0_229ea06f16c9  Operator=mod  SaturateOnIntegerOverflow=on  mask(TL_Math){data={'date',735951.66843344911}}
      settings: CopyFcn=if exist('tl_reset_reviewflag','file')==2,tl_reset_reviewflag(gcbh);end  DeleteFcn=if exist('delete_tlblock','file')==2,delete_tlblock(gcbh);end  NameChangeFcn=if exist('rename_tlblock','file')==2,rename_tlblock(gcbh);end  OpenFcn=if exist('tl_open_blockdlg','file')==2,tl_open_blockdlg(gcbh);else,open_system(gcbh,'parameter');end
      mask Help: eval(['if exist(''tl_online_help'',''file'') == 2, tl_online_help(''Topic'',''TL_Math''),else, web([''jar:file:///'',matlabroot,''/help/toolbox/simulink/help.jar!/slref/' lower(get_param(gcbh,'Blocktype')) '.html''], ''-helpbrowser''),end'])
      mask Display: plot([-0.05, 1.05, NaN, -0.05, 1.05],[.01, .01, NaN, .99, .99])
  Relational Operator1 : RelationalOperator  RequirementInfo={} %GIDa_95bf9cc7_8ac7_4077_bf87_7ecaa1b27c7e  Operator===  OutDataTypeStr=boolean  mask(TL_RelationalOperator){data={'date',735951.66843310185}}
      settings: DeleteFcn=if exist('delete_tlblock','file')==2,delete_tlblock(gcbh);end  NameChangeFcn=if exist('rename_tlblock','file')==2,rename_tlblock(gcbh);end  OpenFcn=if exist('tl_open_blockdlg','file')==2,tl_open_blockdlg(gcbh);else,open_system(gcbh,'parameter');end
      mask Help: eval(['if exist(''tl_online_help'',''file'') == 2, tl_online_help(''Topic'',''TL_RelationalOperator''),else, web([''jar:file:///'',matlabroot,''/help/toolbox/simulink/help.jar!/slref/' lower(get_param(gcbh,'Blocktype')) '.html''], ''-helpbrowser''),end'])
      mask Display: plot([-0.05, 1.05, NaN, -0.05, 1.05],[.01, .01, NaN, .99, .99])
  Sum : Sum  RequirementInfo={} %GIDa_9be2e610_f1b1_4e47_b01f_4b2eb3bde41b  mask(TL_Sum){data={'output',{'type','CONTINUOUS'},'date',735951.66843283561}}
      settings: CopyFcn=if exist('tl_reset_reviewflag','file')==2,tl_reset_reviewflag(gcbh);end  DeleteFcn=if exist('delete_tlblock','file')==2,delete_tlblock(gcbh);end  NameChangeFcn=if exist('rename_tlblock','file')==2,rename_tlblock(gcbh);end  OpenFcn=if exist('tl_open_blockdlg','file')==2,tl_open_blockdlg(gcbh);else,open_system(gcbh,'parameter');end
      mask Help: eval(['if exist(''tl_online_help'',''file'') == 2, tl_online_help(''Topic'',''TL_Sum''),else, web([''jar:file:///'',matlabroot,''/help/toolbox/simulink/help.jar!/slref/' lower(get_param(gcbh,'Blocktype')) '.html''], ''-helpbrowser''),end'])
      mask Display: plot([-0.05, 1.05, NaN, -0.05, 1.05],[.01, .01, NaN, .99, .99])
  Unit Delay : UnitDelay  RequirementInfo={} %GIDa_e0a69db8_f645_4c95_8a6b_4ab4ed108d08  InitialCondition=-1  SampleTime=-1  mask(TL_UnitDelay){data={'date',735951.6684324306}}
      settings: CopyFcn=if exist('tl_reset_reviewflag','file')==2,tl_reset_reviewflag(gcbh);end  DeleteFcn=if exist('delete_tlblock','file')==2,delete_tlblock(gcbh);end  NameChangeFcn=if exist('rename_tlblock','file')==2,rename_tlblock(gcbh);end  OpenFcn=if exist('tl_open_blockdlg','file')==2,tl_open_blockdlg(gcbh);else,open_system(gcbh,'parameter');end
      mask Help: eval(['if exist(''tl_online_help'',''file'') == 2, tl_online_help(''Topic'',''TL_UnitDelay''),else, web([''jar:file:///'',matlabroot,''/help/toolbox/simulink/help.jar!/slref/' lower(get_param(gcbh,'Blocktype')) '.html''], ''-helpbrowser''),end'])
      mask Display: plot([-0.05, 1.05, NaN, -0.05, 1.05],[.01, .01, NaN, .99, .99])
  Out1 : Outport  RequirementInfo={} %GIDa_458d795a_c571_4119_a0fd_b017a19ce0fb
  wires:
  Constant/1 -> Sum/1
  Unit Delay/1 -> Sum/2
  Sum/1 -> Unit Delay/1, Math1/1
  Constant2/1 -> Math1/2
  Math1/1 -> Relational Operator1/1
  Constant4/1 -> Relational Operator1/2
  If/1 -> If Action Subsystem/Action
  If Action Subsystem/1(Out1) -> Out1/1
  Relational Operator1/1 -> If/1

== system BFE_TestHarness/BFE_AC_BeltFunctionExecution/Subsystem/BFE_AC_BeltFunctionExecution/BFE_AC_BeltFunctionExecution/ManageRunnables/If Action Subsystem1 ==
  Trigger : TriggerPort  RequirementInfo={} %GIDa_47eeeb22_0c74_4129_83a9_9fde4f04e822  TriggerType=function-call
  Constant5 : Constant  RequirementInfo={} %GIDa_fe50991d_fd3f_437a_94c5_2722871452dc  mask(TL_Constant){data={'date',735951.66843194445}}
      settings: CopyFcn=if exist('tl_reset_reviewflag','file')==2,tl_reset_reviewflag(gcbh);end  DeleteFcn=if exist('delete_tlblock','file')==2,delete_tlblock(gcbh);end  NameChangeFcn=if exist('rename_tlblock','file')==2,rename_tlblock(gcbh);end  OpenFcn=if exist('tl_open_blockdlg','file')==2,tl_open_blockdlg(gcbh);else,open_system(gcbh,'parameter');end
      mask Help: eval(['if exist(''tl_online_help'',''file'') == 2, tl_online_help(''Topic'',''TL_Constant''),else, web([''jar:file:///'',matlabroot,''/help/toolbox/simulink/help.jar!/slref/' lower(get_param(gcbh,'Blocktype')) '.html''], ''-helpbrowser''),end'])
      mask Display: plot([-0.05, 1.05, NaN, -0.05, 1.05],[.01, .01, NaN, .99, .99])
  Constant6 : Constant  RequirementInfo={} %GIDa_e94159bf_0cec_4118_81bb_87ba086fa164  Value=5  mask(TL_Constant){data={'date',735951.66843157413}}
      settings: CopyFcn=if exist('tl_reset_reviewflag','file')==2,tl_reset_reviewflag(gcbh);end  DeleteFcn=if exist('delete_tlblock','file')==2,delete_tlblock(gcbh);end  NameChangeFcn=if exist('rename_tlblock','file')==2,rename_tlblock(gcbh);end  OpenFcn=if exist('tl_open_blockdlg','file')==2,tl_open_blockdlg(gcbh);else,open_system(gcbh,'parameter');end
      mask Help: eval(['if exist(''tl_online_help'',''file'') == 2, tl_online_help(''Topic'',''TL_Constant''),else, web([''jar:file:///'',matlabroot,''/help/toolbox/simulink/help.jar!/slref/' lower(get_param(gcbh,'Blocktype')) '.html''], ''-helpbrowser''),end'])
      mask Display: plot([-0.05, 1.05, NaN, -0.05, 1.05],[.01, .01, NaN, .99, .99])
  Constant8 : Constant  RequirementInfo={} %GIDa_9e4b394e_f2ab_4111_aa5f_aa3d132fc047  Value=0  mask(TL_Constant){data={'date',735951.66843121522}}
      settings: CopyFcn=if exist('tl_reset_reviewflag','file')==2,tl_reset_reviewflag(gcbh);end  DeleteFcn=if exist('delete_tlblock','file')==2,delete_tlblock(gcbh);end  NameChangeFcn=if exist('rename_tlblock','file')==2,rename_tlblock(gcbh);end  OpenFcn=if exist('tl_open_blockdlg','file')==2,tl_open_blockdlg(gcbh);else,open_system(gcbh,'parameter');end
      mask Help: eval(['if exist(''tl_online_help'',''file'') == 2, tl_online_help(''Topic'',''TL_Constant''),else, web([''jar:file:///'',matlabroot,''/help/toolbox/simulink/help.jar!/slref/' lower(get_param(gcbh,'Blocktype')) '.html''], ''-helpbrowser''),end'])
      mask Display: plot([-0.05, 1.05, NaN, -0.05, 1.05],[.01, .01, NaN, .99, .99])
  If : If  RequirementInfo={} %GIDa_043172a4_6ca5_4414_b8ec_a6f87c755dba  IfExpression=u1  ShowElse=off
  If Action Subsystem : Subsystem  RequirementInfo={} %GIDa_5c201403_5ea9_4e0b_91fd_a798a6177e74  TreatAsAtomicUnit=on
  Math2 : Math  RequirementInfo={} %GIDa_21f38737_0b8b_42e6_a98b_ecfde6ec2765  Operator=mod  SaturateOnIntegerOverflow=on  mask(TL_Math){data={'date',735951.66843082174}}
      settings: CopyFcn=if exist('tl_reset_reviewflag','file')==2,tl_reset_reviewflag(gcbh);end  DeleteFcn=if exist('delete_tlblock','file')==2,delete_tlblock(gcbh);end  NameChangeFcn=if exist('rename_tlblock','file')==2,rename_tlblock(gcbh);end  OpenFcn=if exist('tl_open_blockdlg','file')==2,tl_open_blockdlg(gcbh);else,open_system(gcbh,'parameter');end
      mask Help: eval(['if exist(''tl_online_help'',''file'') == 2, tl_online_help(''Topic'',''TL_Math''),else, web([''jar:file:///'',matlabroot,''/help/toolbox/simulink/help.jar!/slref/' lower(get_param(gcbh,'Blocktype')) '.html''], ''-helpbrowser''),end'])
      mask Display: plot([-0.05, 1.05, NaN, -0.05, 1.05],[.01, .01, NaN, .99, .99])
  Relational Operator2 : RelationalOperator  RequirementInfo={} %GIDa_0a60ef90_36ba_4e0d_8eb0_b50c2dced508  Operator===  OutDataTypeStr=boolean  mask(TL_RelationalOperator){data={'date',735951.66843013884}}
      settings: DeleteFcn=if exist('delete_tlblock','file')==2,delete_tlblock(gcbh);end  NameChangeFcn=if exist('rename_tlblock','file')==2,rename_tlblock(gcbh);end  OpenFcn=if exist('tl_open_blockdlg','file')==2,tl_open_blockdlg(gcbh);else,open_system(gcbh,'parameter');end
      mask Help: eval(['if exist(''tl_online_help'',''file'') == 2, tl_online_help(''Topic'',''TL_RelationalOperator''),else, web([''jar:file:///'',matlabroot,''/help/toolbox/simulink/help.jar!/slref/' lower(get_param(gcbh,'Blocktype')) '.html''], ''-helpbrowser''),end'])
      mask Display: plot([-0.05, 1.05, NaN, -0.05, 1.05],[.01, .01, NaN, .99, .99])
  Scope : Scope
      settings: RequirementInfo={} %GIDa_2804a775_692e_4c53_a90e_836b8f9ecab7
  Sum1 : Sum  RequirementInfo={} %GIDa_a88c1b60_68d2_44e0_9ebb_ae2046e7ca2a  mask(TL_Sum){data={'output',{'type','CONTINUOUS'},'date',735951.66842987272}}
      settings: CopyFcn=if exist('tl_reset_reviewflag','file')==2,tl_reset_reviewflag(gcbh);end  DeleteFcn=if exist('delete_tlblock','file')==2,delete_tlblock(gcbh);end  NameChangeFcn=if exist('rename_tlblock','file')==2,rename_tlblock(gcbh);end  OpenFcn=if exist('tl_open_blockdlg','file')==2,tl_open_blockdlg(gcbh);else,open_system(gcbh,'parameter');end
      mask Help: eval(['if exist(''tl_online_help'',''file'') == 2, tl_online_help(''Topic'',''TL_Sum''),else, web([''jar:file:///'',matlabroot,''/help/toolbox/simulink/help.jar!/slref/' lower(get_param(gcbh,'Blocktype')) '.html''], ''-helpbrowser''),end'])
      mask Display: plot([-0.05, 1.05, NaN, -0.05, 1.05],[.01, .01, NaN, .99, .99])
  Unit Delay1 : UnitDelay  RequirementInfo={} %GIDa_12a13dff_a6da_4003_85ff_ebd809442c72  InitialCondition=-1  SampleTime=-1  mask(TL_UnitDelay){data={'date',735951.66842946759}}
      settings: CopyFcn=if exist('tl_reset_reviewflag','file')==2,tl_reset_reviewflag(gcbh);end  DeleteFcn=if exist('delete_tlblock','file')==2,delete_tlblock(gcbh);end  NameChangeFcn=if exist('rename_tlblock','file')==2,rename_tlblock(gcbh);end  OpenFcn=if exist('tl_open_blockdlg','file')==2,tl_open_blockdlg(gcbh);else,open_system(gcbh,'parameter');end
      mask Help: eval(['if exist(''tl_online_help'',''file'') == 2, tl_online_help(''Topic'',''TL_UnitDelay''),else, web([''jar:file:///'',matlabroot,''/help/toolbox/simulink/help.jar!/slref/' lower(get_param(gcbh,'Blocktype')) '.html''], ''-helpbrowser''),end'])
      mask Display: plot([-0.05, 1.05, NaN, -0.05, 1.05],[.01, .01, NaN, .99, .99])
  Out1 : Outport  RequirementInfo={} %GIDa_28102d3c_0a6c_4e70_99a6_394d6d6e86be
  wires:
  Constant5/1 -> Sum1/1
  Unit Delay1/1 -> Sum1/2
  Sum1/1 -> Unit Delay1/1, Math2/1
  Constant6/1 -> Math2/2
  Math2/1 -> Relational Operator2/2, Scope/1
  Constant8/1 -> Relational Operator2/1
  If/1 -> If Action Subsystem/Action
  Relational Operator2/1 -> If/1
  If Action Subsystem/1(Out1) -> Out1/1
